simulink model "sim_project"  (R2022a)
settings: Solver=FixedStepAuto  StartTime=0.0  StopTime=10.0  FixedStep=0.005  RelTol=1e-3
InitFcn:
  | N = 1;
  | m = 1;
  | l = 0.225;
  | a = 0.1;
  | Icn = 1/3 * (l^2)*N*m + a^2*(N^3)/12;
  | Ixx = 0.0057;
values from neighbouring files (symbols this model uses):
  Is_sim = Is(N)    [momentofinertia.m]    (also in run_sim.m = ureal('Is_sim',Is(N),'Percentage',50); run_sim_N.m; run_sim_uns.m = ureal('Is_sim',Is(N),'Percentage',20))
  K_gain = K_dat(N_sim)    [momentofinertia.m]    (also in run_sim.m = K_dat(N); run_sim_N.m = K_dat(N); run_sim_uns.m = K_dat(N))
  N_sim = 1    [momentofinertia.m]
  uvars = ufind(mdl)    [run_sim.m]    (also in run_sim_uns.m)
undefined symbols (not defined in the file or in its folder): Izz, usample
libraries: slpidlib x3, RCTblocks x2, simulink_extras x2
settings Model: Creator=Kerim  LastModifiedBy=Kerim
settings SolverCC: AlgebraicLoopSolver=TrustRegion
settings DebuggingCC: UnconnectedInputMsg=warning  UnconnectedOutputMsg=warning  UnconnectedLineMsg=warning  SFMachineParentedDataDiag=warning
settings RTWCC: DLArmComputeVersion=19.05

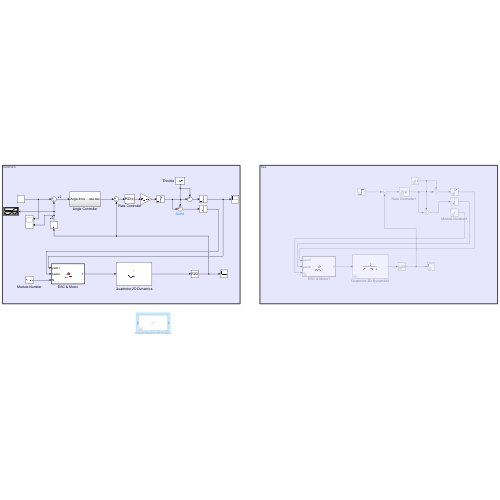
[thumbnail: Simulink's stored preview of the top-level diagram]
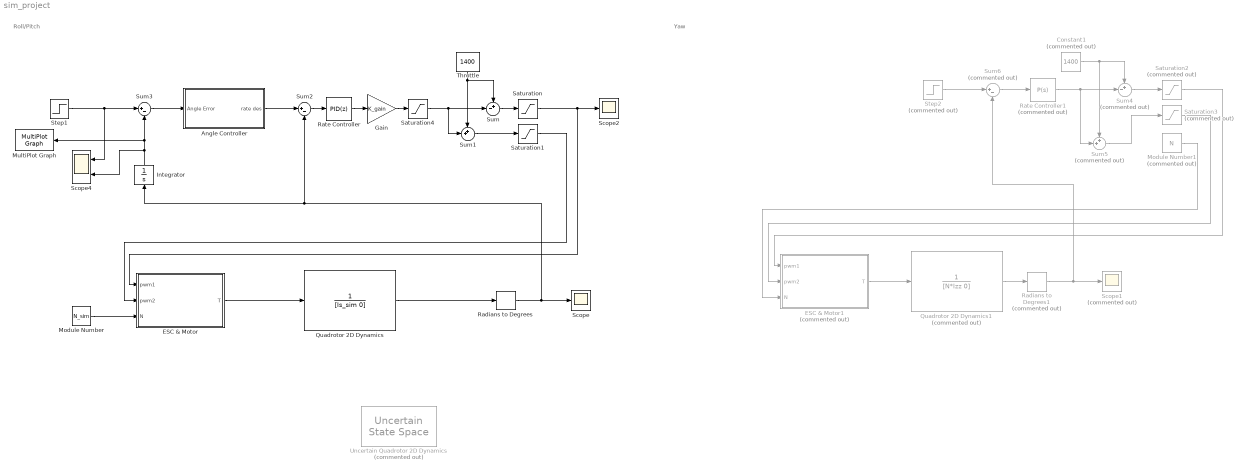
== system sim_project ==
  note: Roll/Pitch
  note: Yaw
  Angle Controller : Subsystem
  Constant1 : Constant  Commented=on  Value=1400
  ESC & Motor : MATLAB Function  TreatAsAtomicUnit=on
  ESC & Motor1 : MATLAB Function  Commented=on  TreatAsAtomicUnit=on
  Gain : Gain  Gain=K_gain
  Integrator : Integrator
  Module Number : Constant  Value=N_sim
  Module Number1 : Constant  Commented=on  Value=N
  MultiPlot Graph : RCTblocks/MultiPlot Graph  Tag=MultiPlot  tmin=0  tmax=10  ymin=-1  ymax=2  Tsamp=-1  vnamesave=multisimout
      settings: SourceProductBaseCode=RC
  Quadrotor 2D Dynamics : TransferFcn  Denominator=[Is_sim 0]
  Quadrotor 2D Dynamics1 : TransferFcn  Commented=on  Denominator=[N*Izz 0]
  Radians to Degrees : simulink_extras/Transformations/Radians to Degrees
  Radians to Degrees1 : simulink_extras/Transformations/Radians to Degrees  Commented=on
  Rate Controller : slpidlib/PID Controller  Controller=PID  Form=Parallel  TimeDomain=Discrete-time  UseExternalTs=off  SampleTime=-1  IntegratorMethod=Forward Euler  FilterMethod=Forward Euler  ControllerParametersSource=internal  P=0.48  I=0.08  UseKiTs=off  D=0.008  N=100  UseFilter=on  TunerSelectOption=Transfer Function Based (PID Tuner App)  InitialConditionSource=internal  InitialConditionForIntegrator=0  InitialConditionForFilter=0  DifferentiatorICPrevScaledInput=0  ExternalReset=none  TrackingMode=off  Kt=1  LimitOutput=off  SatLimitsSource=internal  UpperSaturationLimit=inf  LowerSaturationLimit=-inf  LinearizeAsGain=on  AntiWindupMode=none  Kb=1  POutMin=[]  POutMax=[]  IOutMin=[]  IOutMax=[]  DOutMin=[]  DOutMax=[]  NOutMin=[]  NOutMax=[]  SumOutMin=[]  SumOutMax=[]  SaturationOutMin=[]  SaturationOutMax=[]  PParamMin=[]  PParamMax=[]  IParamMin=[]  IParamMax=[]  DParamMin=[]  DParamMax=[]  NParamMin=[]  NParamMax=[]  KbParamMin=[]  KbParamMax=[]  KtParamMin=[]  KtParamMax=[]  KbOutMin=[]  KbOutMax=[]  KtOutMin=[]  KtOutMax=[]  IntegratorOutMin=[]  IntegratorOutMax=[]  FilterOutMin=[]  FilterOutMax=[]  SumI1OutMin=[]  SumI1OutMax=[]  SumI2OutMin=[]  SumI2OutMax=[]  SumI3OutMin=[]  SumI3OutMax=[]  SumI4OutMin=[]  SumI4OutMax=[]  SumDOutMin=[]  SumDOutMax=[]  DifferentiatorOutMin=[]  DifferentiatorOutMax=[]  FilterDiffOutCoefMin=[]  FilterDiffOutCoefMax=[]  ReciprocalOutMin=[]  ReciprocalOutMax=[]  SumDenOutMin=[]  SumDenOutMax=[]  SumNumOutMin=[]  SumNumOutMax=[]  DivideOutMin=[]  DivideOutMax=[]  UdiffTsProdOutMin=[]  UdiffTsProdOutMax=[]  NTsProdOutMin=[]  NTsProdOutMax=[]  UintegralTsProdOutMin=[]  UintegralTsProdOutMax=[]  UngainTsProdOutMin=[]  UngainTsProdOutMax=[]  IntegratorContinuousStateAttributes=''  IntegratorStateMustResolveToSignalObject=off  IntegratorRTWStateStorageClass=Auto  FilterContinuousStateAttributes=''  FilterStateMustResolveToSignalObject=off  FilterRTWStateStorageClass=Auto  ParallelPVariant=InternalParameters  IdealPVariant=Disabled  IVariant=InternalParameters  DVariant=InternalParameters  IntegratorVariant=Discrete  SatVariant=Disabled  AWVariant=Passthrough  PCopyVariant=Disabled  TRVariant=Disabled  FdbkBlocksVariant=Forward  IdealPFdbkVariant=Disabled  SatFdbkVariant=Disabled  DerivativeFilterVariant=ForwardEulerFilter  NVariant=InternalParameters  NCopyVariant=Disabled  FilterICVariant=InternalICsFilter  IntegratorICVariant=InternalICs  ExternalResetVariant=Disabled  TRSumVariant=Passthrough  SumFdbkVariant=Disabled  SumVariant=Sum_PID  TsampFilterVariant=InternalTs  TsampNgainVariant=Passthrough  TsampIntegralVariant=Passthrough  ExternalSaturationOutDataTypeStr=Inherit: Same as second input  aMode=0
  Rate Controller1 : slpidlib/PID Controller  Commented=on  Controller=P  Form=Parallel  TimeDomain=Continuous-time  UseExternalTs=off  SampleTime=-1  IntegratorMethod=Forward Euler  FilterMethod=Forward Euler  ControllerParametersSource=internal  P=5  I=1  UseKiTs=off  D=K_gain*0.06  N=345.128531237038  UseFilter=on  TunerSelectOption=Transfer Function Based (PID Tuner App)  InitialConditionSource=internal  InitialConditionForIntegrator=0  InitialConditionForFilter=0  DifferentiatorICPrevScaledInput=0  ExternalReset=none  TrackingMode=off  Kt=1  LimitOutput=off  SatLimitsSource=internal  UpperSaturationLimit=inf  LowerSaturationLimit=-inf  LinearizeAsGain=on  AntiWindupMode=none  Kb=1  POutMin=[]  POutMax=[]  IOutMin=[]  IOutMax=[]  DOutMin=[]  DOutMax=[]  NOutMin=[]  NOutMax=[]  SumOutMin=[]  SumOutMax=[]  SaturationOutMin=[]  SaturationOutMax=[]  PParamMin=[]  PParamMax=[]  IParamMin=[]  IParamMax=[]  DParamMin=[]  DParamMax=[]  NParamMin=[]  NParamMax=[]  KbParamMin=[]  KbParamMax=[]  KtParamMin=[]  KtParamMax=[]  KbOutMin=[]  KbOutMax=[]  KtOutMin=[]  KtOutMax=[]  IntegratorOutMin=[]  IntegratorOutMax=[]  FilterOutMin=[]  FilterOutMax=[]  SumI1OutMin=[]  SumI1OutMax=[]  SumI2OutMin=[]  SumI2OutMax=[]  SumI3OutMin=[]  SumI3OutMax=[]  SumI4OutMin=[]  SumI4OutMax=[]  SumDOutMin=[]  SumDOutMax=[]  DifferentiatorOutMin=[]  DifferentiatorOutMax=[]  FilterDiffOutCoefMin=[]  FilterDiffOutCoefMax=[]  ReciprocalOutMin=[]  ReciprocalOutMax=[]  SumDenOutMin=[]  SumDenOutMax=[]  SumNumOutMin=[]  SumNumOutMax=[]  DivideOutMin=[]  DivideOutMax=[]  UdiffTsProdOutMin=[]  UdiffTsProdOutMax=[]  NTsProdOutMin=[]  NTsProdOutMax=[]  UintegralTsProdOutMin=[]  UintegralTsProdOutMax=[]  UngainTsProdOutMin=[]  UngainTsProdOutMax=[]  IntegratorContinuousStateAttributes=''  IntegratorStateMustResolveToSignalObject=off  IntegratorRTWStateStorageClass=Auto  FilterContinuousStateAttributes=''  FilterStateMustResolveToSignalObject=off  FilterRTWStateStorageClass=Auto  ParallelPVariant=InternalParameters  IdealPVariant=Disabled  IVariant=Disabled  DVariant=Disabled  IntegratorVariant=Disabled  SatVariant=Disabled  AWVariant=Disabled  PCopyVariant=Disabled  TRVariant=Disabled  FdbkBlocksVariant=Forward  IdealPFdbkVariant=Disabled  SatFdbkVariant=Disabled  DerivativeFilterVariant=Disabled  NVariant=Disabled  NCopyVariant=Disabled_SignalSpec  FilterICVariant=Disabled  IntegratorICVariant=Disabled  ExternalResetVariant=Disabled  TRSumVariant=Passthrough  SumFdbkVariant=Disabled  SumVariant=Passthrough_P  TsampFilterVariant=InternalTs  TsampNgainVariant=Passthrough  TsampIntegralVariant=Disabled_SignalSpec  ExternalSaturationOutDataTypeStr=Inherit: Same as second input  aMode=0
  Saturation : Saturate  UpperLimit=1900  LowerLimit=1100
  Saturation1 : Saturate  UpperLimit=1900  LowerLimit=1100
  Saturation2 : Saturate  Commented=on  UpperLimit=1900  LowerLimit=1100
  Saturation3 : Saturate  Commented=on  UpperLimit=1900  LowerLimit=1100
  Saturation4 : Saturate  UpperLimit=300  LowerLimit=-300
  Scope : Scope
  Scope1 : Scope  Commented=on
  Scope2 : Scope
  Scope4 : Scope  NumInputPorts=2
  Step1 : Step  SampleTime=0
  Step2 : Step  Commented=on  SampleTime=0
  Sum : Sum  Inputs=+-|
  Sum1 : Sum  Inputs=++|
  Sum2 : Sum  Inputs=|+-
  Sum3 : Sum  Inputs=|+-
  Sum4 : Sum  Commented=on  Inputs=+-|
  Sum5 : Sum  Commented=on  Inputs=++|
  Sum6 : Sum  Commented=on  Inputs=|+-
  Throttle : Constant  Value=1400
  Uncertain Quadrotor 2D Dynamics : RCTblocks/Uncertain State Space  Tag=USS  Commented=on  USystem=usys  UValue=usample(uvars)  X0=[]  uX0=[]
      settings: SourceProductBaseCode=RC
  wires:
  Rate Controller/1 -> Gain/1
  Throttle/1 -> Sum/1, Sum1/1
  Angle Controller/1(rate des) -> Sum2/1
  Saturation/1 -> Scope2/1, ESC & Motor/1(pwm1)
  Sum/1 -> Saturation/1
  Saturation1/1 -> ESC & Motor/2(pwm2)
  Sum1/1 -> Saturation1/1
  Sum2/1 -> Rate Controller/1
  Module Number/1 -> ESC & Motor/3(N)
  Sum3/1 -> Angle Controller/1(Angle Error)
  Step1/1 -> Scope4/1, Sum3/1
  Quadrotor 2D Dynamics1/1 -> Radians to Degrees1/1
  Rate Controller1/1 -> Sum5/2, Sum4/2
  Sum5/1 -> Saturation3/1
  Sum6/1 -> Rate Controller1/1
  Module Number1/1 -> ESC & Motor1/3(N)
  Saturation3/1 -> ESC & Motor1/2(pwm2)
  Saturation2/1 -> ESC & Motor1/1(pwm1)
  ESC & Motor1/1(T) -> Quadrotor 2D Dynamics1/1
  Constant1/1 -> Sum5/1, Sum4/1
  Sum4/1 -> Saturation2/1
  Radians to Degrees1/1 -> Sum6/2, Scope1/1
  Step2/1 -> Sum6/1
  Radians to Degrees/1 -> Scope/1, Sum2/2, Integrator/1
  Integrator/1 -> Scope4/2, Sum3/2, MultiPlot Graph/1
  Gain/1 -> Saturation4/1
  Saturation4/1 -> Sum1/2, Sum/2
  ESC & Motor/1(T) -> Quadrotor 2D Dynamics/1
  Quadrotor 2D Dynamics/1 -> Radians to Degrees/1

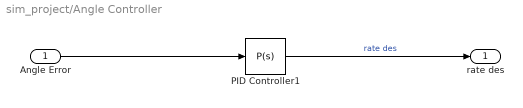
== system sim_project/Angle Controller ==
  Angle Error : Inport
  PID Controller1 : slpidlib/PID Controller  Controller=P  Form=Parallel  TimeDomain=Continuous-time  UseExternalTs=off  SampleTime=-1  IntegratorMethod=Forward Euler  FilterMethod=Forward Euler  ControllerParametersSource=internal  P=4.5  I=0  UseKiTs=off  D=0  N=100  UseFilter=on  TunerSelectOption=Transfer Function Based (PID Tuner App)  InitialConditionSource=internal  InitialConditionForIntegrator=0  InitialConditionForFilter=0  DifferentiatorICPrevScaledInput=0  ExternalReset=none  TrackingMode=off  Kt=1  LimitOutput=off  SatLimitsSource=internal  UpperSaturationLimit=inf  LowerSaturationLimit=-inf  LinearizeAsGain=on  AntiWindupMode=none  Kb=1  POutMin=[]  POutMax=[]  IOutMin=[]  IOutMax=[]  DOutMin=[]  DOutMax=[]  NOutMin=[]  NOutMax=[]  SumOutMin=[]  SumOutMax=[]  SaturationOutMin=[]  SaturationOutMax=[]  PParamMin=[]  PParamMax=[]  IParamMin=[]  IParamMax=[]  DParamMin=[]  DParamMax=[]  NParamMin=[]  NParamMax=[]  KbParamMin=[]  KbParamMax=[]  KtParamMin=[]  KtParamMax=[]  KbOutMin=[]  KbOutMax=[]  KtOutMin=[]  KtOutMax=[]  IntegratorOutMin=[]  IntegratorOutMax=[]  FilterOutMin=[]  FilterOutMax=[]  SumI1OutMin=[]  SumI1OutMax=[]  SumI2OutMin=[]  SumI2OutMax=[]  SumI3OutMin=[]  SumI3OutMax=[]  SumI4OutMin=[]  SumI4OutMax=[]  SumDOutMin=[]  SumDOutMax=[]  DifferentiatorOutMin=[]  DifferentiatorOutMax=[]  FilterDiffOutCoefMin=[]  FilterDiffOutCoefMax=[]  ReciprocalOutMin=[]  ReciprocalOutMax=[]  SumDenOutMin=[]  SumDenOutMax=[]  SumNumOutMin=[]  SumNumOutMax=[]  DivideOutMin=[]  DivideOutMax=[]  UdiffTsProdOutMin=[]  UdiffTsProdOutMax=[]  NTsProdOutMin=[]  NTsProdOutMax=[]  UintegralTsProdOutMin=[]  UintegralTsProdOutMax=[]  UngainTsProdOutMin=[]  UngainTsProdOutMax=[]  IntegratorContinuousStateAttributes=''  IntegratorStateMustResolveToSignalObject=off  IntegratorRTWStateStorageClass=Auto  FilterContinuousStateAttributes=''  FilterStateMustResolveToSignalObject=off  FilterRTWStateStorageClass=Auto  ParallelPVariant=InternalParameters  IdealPVariant=Disabled  IVariant=Disabled  DVariant=Disabled  IntegratorVariant=Disabled  SatVariant=Disabled  AWVariant=Disabled  PCopyVariant=Disabled  TRVariant=Disabled  FdbkBlocksVariant=Forward  IdealPFdbkVariant=Disabled  SatFdbkVariant=Disabled  DerivativeFilterVariant=Disabled  NVariant=Disabled  NCopyVariant=Disabled_SignalSpec  FilterICVariant=Disabled  IntegratorICVariant=Disabled  ExternalResetVariant=Disabled  TRSumVariant=Passthrough  SumFdbkVariant=Disabled  SumVariant=Passthrough_P  TsampFilterVariant=InternalTs  TsampNgainVariant=Passthrough  TsampIntegralVariant=Disabled_SignalSpec  ExternalSaturationOutDataTypeStr=Inherit: Same as second input  aMode=0
  rate des : Outport
  wires:
  Angle Error/1 -> PID Controller1/1
  PID Controller1/1 -> rate des/1  "rate des"

== matlab function sim_project/ESC & Motor1 ==
  data: pwm1 input; T output; pwm2 input; N input
function T = pwm2T(pwm1,pwm2,N)
max_thrust = 940/1000 * 10;
max_rpm = 13610;
k = max_thrust / (max_rpm^2)*0.05;
l = 0.15;
w1 = (pwm1 - 1000) * (max_rpm - 0) / (2000 - 1000) + 0;
w2 = (pwm2 - 1000) * (max_rpm - 0) / (2000 - 1000) + 0;


M1 = k*w1^2; M2=k*w2^2;

T = N*2*(M2-M1);

== matlab function sim_project/ESC & Motor ==
  data: pwm1 input; T output; pwm2 input; N input
function T = pwm2T(pwm1,pwm2,N)
max_thrust = 940/1000 * 10;
max_rpm = 13610;
k = max_thrust / (max_rpm^2);
l = 0.2;
w1 = (pwm1 - 1000) * (max_rpm - 0) / (2000 - 1000) + 0;
w2 = (pwm2 - 1000) * (max_rpm - 0) / (2000 - 1000) + 0;


F1 = k*w1^2; F2=k*w2^2;

T = N*2*(F2-F1)*l;
